simulink model "low"  (R2014a)
settings: Solver=FixedStepDiscrete  StartTime=0.0  StopTime=SimLength  FixedStep=sample_time  RelTol=1e-3
undefined symbols (not defined in the file): SimLength
libraries: simulink x3, dspswit3 x1
settings Model: Creator=Maik  LastModifiedBy=Maik

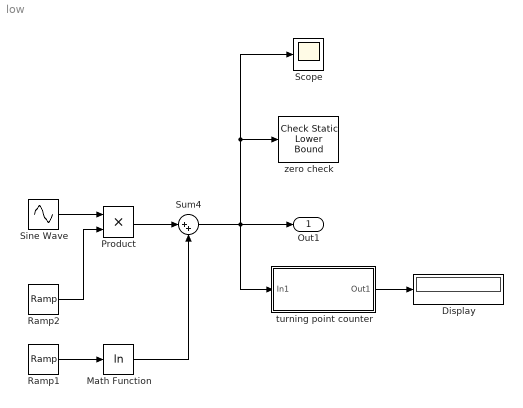
== system low ==
  Display : Display
  Math Function : Math  Operator=log  SaturateOnIntegerOverflow=on
  Product : Product
  Ramp1 : simulink/Sources/Ramp  slope=1  start=0  X0=1
  Ramp2 : simulink/Sources/Ramp  slope=1/SimLength  start=0  X0=0
  Scope : Scope
      settings: YMin=-1  YMax=1  SaveName=ScopeData5
  Sine Wave : Sin  Amplitude=0.3  Frequency=0.5
  Sum4 : Sum  Inputs=|++
  turning point counter : Subsystem
  zero check : simulink/Model Verification/Check Static  Lower Bound  Description=0 <= u  min=0  min_included=on  enabled=on  stopWhenAssertionFail=on  export=off  icon=text
  Out1 : Outport
  wires:
  turning point counter/1(Out1) -> Display/1
  Math Function/1 -> Sum4/2
  Ramp1/1 -> Math Function/1
  Ramp2/1 -> Product/2
  Sine Wave/1 -> Product/1
  Product/1 -> Sum4/1
  Sum4/1 -> turning point counter/1(In1), Scope/1, zero check/1, Out1/1

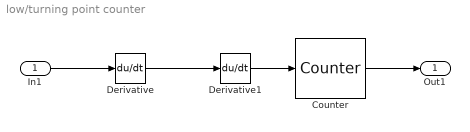
== system low/turning point counter ==
  In1 : Inport
  Counter : dspswit3/Counter  Direction=Up  CountEvent=Either edge  CounterSize=16 bits  MaxCount=255  InitialCount=0  Output=Count  HitValue=0  ResetInput=off  SamplesPerFrame=1  Ts=1  CntDtype=single  HitDtype=Logical
  Derivative : Derivative
  Derivative1 : Derivative
  Out1 : Outport
  wires:
  In1/1 -> Derivative/1
  Derivative/1 -> Derivative1/1
  Derivative1/1 -> Counter/1
  Counter/1 -> Out1/1
